simulink model "Test1MotorEnterMotorMode"  (R2023b)
settings: Solver=FixedStepAuto  StartTime=0.0  StopTime=inf  RelTol=1e-3  EnableMultiTasking=on
model workspace (MAT data in the model file):
  Can_ID = 0
libraries: canmsglib x3, arduinolib x3
settings Model: ExtModeTrigDuration=2  Creator=Antonio  LastModifiedBy=Antonio
settings OptimizationCC: EnhancedBackFolding=on  PassReuseOutputArgsAs=Individual arguments  ZeroExternalMemoryAtStartup=off  ZeroInternalMemoryAtStartup=off  MaxStackSize=64  OptimizeBlockOrder=speed  DifferentSizesBufferReuse=on  OptimizationCustomize=off  EfficientTunableParamExpr=on
settings DebuggingCC: ParameterTunabilityLossMsg=error
settings HardwareCC: ProdBitPerPointer=32  ProdBitPerSizeT=32  ProdBitPerPtrDiffT=32  ProdLargestAtomicInteger=Long  ProdLargestAtomicFloat=Double  ProdWordSize=32  ProdHWDeviceType=ARM Compatible->ARM Cortex
settings SFSimCC: MATLABDynamicMemAlloc=off
settings RTWCC: Description=Embedded Coder  SystemTargetFile=ert.tlc  HardwareBoard=Arduino MKR WiFi 1010  TemplateMakefile=ert_default_tmf  Toolchain=Arduino ARM  BuildConfiguration=Faster Runs
settings CodeAppCC: ForceParamTrailComments=on  IgnoreCustomStorageClasses=off  OperatorAnnotations=on  SimulinkDataObjDesc=on  SFDataObjDesc=on  InsertBlockDesc=on
settings ERTTargetCC: SupportContinuousTime=on  SupportVariableSizeSignals=on  ExtModeTransport=3  ExtModeStaticAlloc=on  ExtModeAutomaticAllocSize=off  ExtModeStaticAllocSize=8192  ExtModeMexFile=ext_xcp  ExtModeIntrfLevel=Level2 - Open

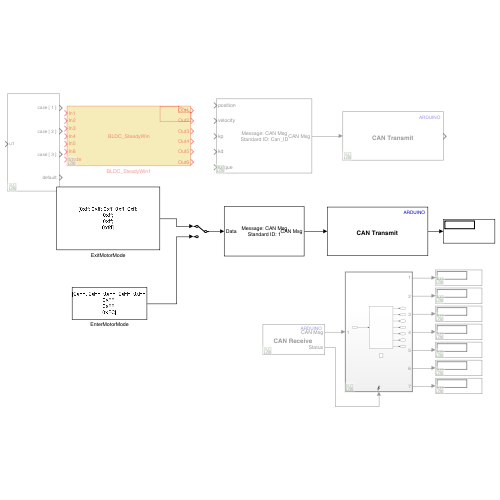
[thumbnail: Simulink's stored preview of the top-level diagram]
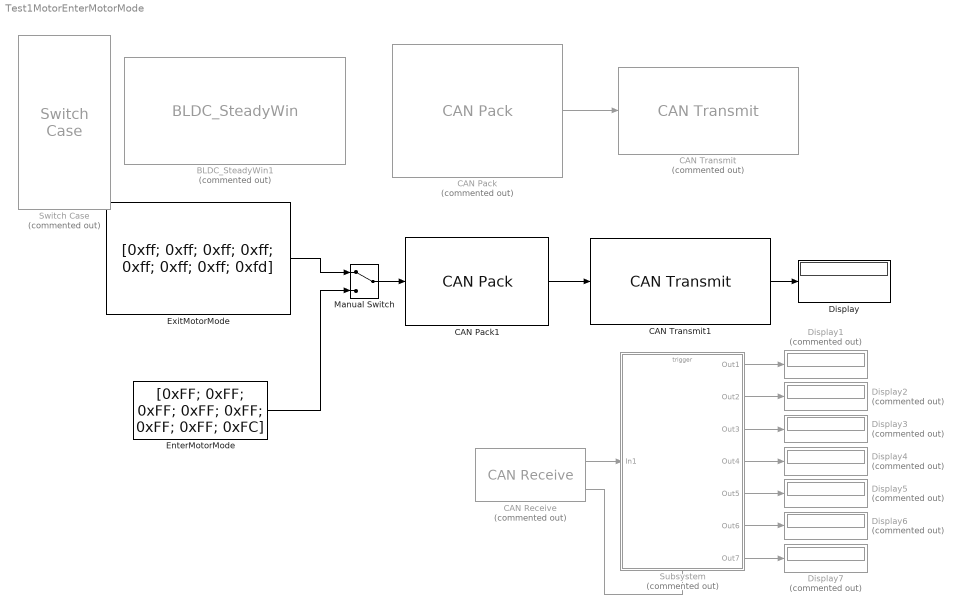
== system Test1MotorEnterMotorMode ==
  BLDC_SteadyWin1 : S-Function  Commented=on  InitFcn=try, set_param(gcb,'FunctionName','BLDC_SteadyWin'), end  FunctionName=BLDC_SteadyWin  SFunctionModules=BLDC_SteadyWinPack_wrapper.cpp  SFunctionDeploymentMode=off  EnableBusSupport=off  mask(S-Function Builder){}
      mask help: Simulink:masks:SFunctionBuilder_MD
      mask init:
      | val = [[.9  0.75 0.75 1 1 .9 .9 1]',[1 1 0.75 0.75 .9 .9 1 .9]'];try , sys = get_param(gcb,'SfunBuilderFcnName');if isempty(sys), sys = get_param(gcb,'FunctionName'); end,catch, sys = get_param(gcb,'FunctionName'); end
      settings: CopyFcn=set_param(gcbh,'LinkStatus','none')  PreSaveFcn=try, set_param(gcb,'FunctionName','BLDC_SteadyWin'), end  OpenFcn=sfunctionwizard(gcbh)
      mask Display:
      | plot(val(:,1),val(:,2))
      | disp(sys)
      | port_label('input',1,'In1')
      | port_label('input',2,'In2')
      | port_label('input',3,'In3')
      | port_label('input',4,'In4')
      | port_label('input',5,'In5')
      | port_label('input',6,'In6')
      | port_label('input',7,'Mode')
      | port_label('output',1,'Out1')
      | port_label('output',2,'Out2')
      | port_label('output',3,'Out3')
      | port_label('output',4,'Out4')
      | port_label('output',5,'Out5')
      | port_label('output',6,'Out6')
  CAN Pack : canmsglib/CAN Pack  Commented=on  MsgList=(none)  MsgName=CAN Msg  MsgIDType=Standard (11-bit identifier)  MsgIdentifier=Can_ID  MsgLength=8  Remote=off  ApplyMinMax=off  BusOutput=off  SignalInfo={ 'position', '8', '16', 'BE', 'signed', 'Standard', '0', '1', '-95.5', '-95.5', '95.5'; 'velocity', '28', '12', 'BE', 'signed', 'Standard', '0', '1', '-45', '-45', '45'; 'kp', '32', '12', 'BE', 'unsigned', 'Standard', '0', '1', '0', '0', '500'; 'kd', '52', '12', 'BE', 'unsigned', 'Standard', '0', '1', '0', '0', '5'; 'torque', '56', '12', 'BE', 'signed', 'Standard', '0', '1', '-18', '-18', '18' }
      settings: LibrarySourceBlock=embeddedtargetslib/Host Communication/CAN Pack  DataFormat=manually specified signals
  CAN Pack1 : canmsglib/CAN Pack  MsgList=(none)  MsgName=CAN Msg  MsgIDType=Standard (11-bit identifier)  MsgIdentifier=1  MsgLength=8  Remote=off  ApplyMinMax=off  BusOutput=on  SignalInfo={ 'position', '8', '16', 'BE', 'signed', 'Standard', '0', '1', '-95.5', '-95.5', '95.5'; 'velocity', '28', '12', 'BE', 'signed', 'Standard', '0', '1', '-45', '-45', '45'; 'kp', '32', '12', 'BE', 'unsigned', 'Standard', '0', '1', '0', '0', '500'; 'kd', '52', '12', 'BE', 'unsigned', 'Standard', '0', '1', '0', '0', '5'; 'torque', '56', '12', 'BE', 'signed', 'Standard', '0', '1', '-18', '-18', '18' }
      settings: LibrarySourceBlock=embeddedtargetslib/Host Communication/CAN Pack  DataFormat=raw data
  CAN Receive : arduinolib/CAN Receive  Commented=on  outputDataType=CAN Msg  identifierType=Standard (11-bit identifier)  messageId=100  msgLength=8  SampleTime=0.1  outputError=off  outputRemote=off
  CAN Transmit : arduinolib/CAN Transmit  Commented=on  inputDataType=CAN Msg  BlockingMode_=on  BlockTimeout_=1  outputStatus=on  identifierType=Standard (11-bit identifier)  messageId=100  msgLength=8  remoteFrame=off
  CAN Transmit1 : arduinolib/CAN Transmit  inputDataType=CAN Msg  BlockingMode_=on  BlockTimeout_=1  outputStatus=on  identifierType=Standard (11-bit identifier)  messageId=100  msgLength=8  remoteFrame=off
  Display : Display
  Display{1..7} (7 alike) : Display  Commented=on
  EnterMotorMode : Constant  Value=|  OutDataTypeStr=uint8
      | [0xFF; 0xFF; 0xFF; 0xFF; 0xFF;
      | 0xFF;
      | 0xFF;
      | 0xFC]
  ExitMotorMode : Constant  Value=|  OutDataTypeStr=uint8
      | [0xff; 0xff; 0xff; 0xff; 0xff;
      | 0xff;
      | 0xff;
      | 0xfd]
  Manual Switch : ManualSwitch
  Subsystem : Subsystem  Commented=on
  Switch Case : SwitchCase  Commented=on  CaseConditions={1 2 3}
  wires:
  CAN Pack/1 -> CAN Transmit/1
  ExitMotorMode/1 -> Manual Switch/1
  EnterMotorMode/1 -> Manual Switch/2
  CAN Pack1/1 -> CAN Transmit1/1
  Manual Switch/1 -> CAN Pack1/1
  CAN Transmit1/1 -> Display/1
  CAN Receive/1 -> Subsystem/1(In1)
  Subsystem/1(Out1) -> Display1/1
  Subsystem/2(Out2) -> Display2/1
  Subsystem/3(Out3) -> Display3/1
  Subsystem/4(Out4) -> Display4/1
  Subsystem/5(Out5) -> Display5/1
  Subsystem/6(Out6) -> Display6/1
  Subsystem/7(Out7) -> Display7/1
  CAN Receive/2 -> Subsystem/Trigger

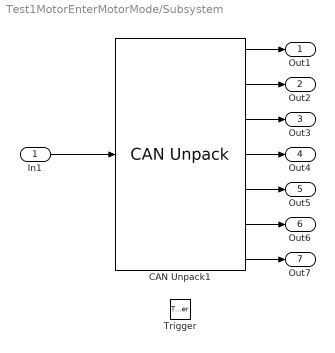
== system Test1MotorEnterMotorMode/Subsystem ==
  In1 : Inport
  Trigger : TriggerPort  VariantControl=(inherit)  PortDimensions=1
  CAN Unpack1 : canmsglib/CAN Unpack  MsgList=(none)  MsgName=CAN Msg  MsgIDType=Standard (11-bit identifier)  MsgIdentifier=1  MsgLength=5  SignalInfo={ 'position', '8', '16', 'BE', 'signed', 'Standard', '0', '343.11518324607329842931937172775', '-95.5', '-95.5', '95.5'; 'velocity', '28', '12', 'BE', 'signed', 'Standard', '0', '45.5', '-45', '-45', '45'; 'current', '32', '12', 'BE', 'signed', 'Standard', '0', '113.75', '-18', '-18', '18' }  IDPort=on  TimestampPort=on  ErrorPort=on  RemotePort=off  LengthPort=off  StatusPort=on  ApplyMinMax=off
      settings: LibrarySourceBlock=embeddedtargetslib/Host Communication/CAN Unpack
  Out1 : Outport
  Out2 : Outport  Port=2
  Out3 : Outport  Port=3
  Out4 : Outport  Port=4
  Out5 : Outport  Port=5
  Out6 : Outport  Port=6
  Out7 : Outport  Port=7
  wires:
  CAN Unpack1/2 -> Out2/1
  CAN Unpack1/7 -> Out7/1
  In1/1 -> CAN Unpack1/1
  CAN Unpack1/5 -> Out5/1
  CAN Unpack1/4 -> Out4/1
  CAN Unpack1/1 -> Out1/1
  CAN Unpack1/6 -> Out6/1
  CAN Unpack1/3 -> Out3/1
